simulink model "lateralForceEstimator"  (R2015b)
settings: Solver=FixedStepAuto  StartTime=0.0  StopTime=1.0  FixedStep=0.001  RelTol=1e-3
values from neighbouring files (symbols this model uses):
  Iz = 4605    [ecs.m]
  lf = 1.141    [ecs.m]
  lr = 1.639    [ecs.m]
  mv = 1529.98    [ecs.m]
undefined symbols (not defined in the file or in its folder): d
libraries: simulink x2
settings Model: Creator=ADMIN  LastModifiedBy=ADMIN

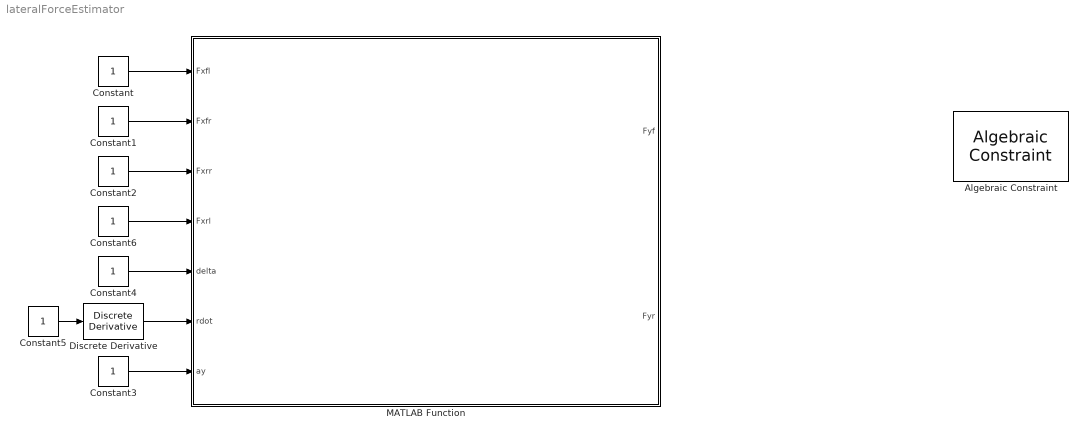
== system lateralForceEstimator ==
  Algebraic Constraint : simulink/Math Operations/Algebraic Constraint  z0=0
  Constant{,1..6} (7 alike) : Constant
  Discrete Derivative : simulink/Discrete/Discrete Derivative  gainval=1.0  ICPrevScaledInput=0.0  InputProcessing=Inherited  OutMin=[]  OutMax=[]  OutDataType=fixdt(1, 16)  OutScaling=2^-10  DoSatur=off
  MATLAB Function : MATLAB Function  InitFcn=|  TreatAsAtomicUnit=on
      | d = 1.795;
      | mv= 1529.98;
      | lf = 1.35;
      | lr = 1.23;
      | Iz = 4605;
  wires:
  Constant/1 -> MATLAB Function/1(Fxfl)
  Constant1/1 -> MATLAB Function/2(Fxfr)
  Constant2/1 -> MATLAB Function/3(Fxrr)
  Constant6/1 -> MATLAB Function/4(Fxrl)
  Constant4/1 -> MATLAB Function/5(delta)
  Constant3/1 -> MATLAB Function/7(ay)
  Constant5/1 -> Discrete Derivative/1
  Discrete Derivative/1 -> MATLAB Function/6(rdot)

== matlab function lateralForceEstimator/MATLAB Function ==
  data: Fxfl input; Fyf output; Fxfr input; Fxrr input; Fxrl input; delta input; rdot input; ay input; Fyr output; d parameter; mv parameter; Iz parameter; lr parameter; lf parameter
function [Fyf, Fyr]= fcn(Fxfl, Fxfr, Fxrr, Fxrl, delta, rdot, ay, d, mv, Iz, lr, lf)
% %#codegen
coder.extrinsic('syms');
syms Fyfs;
syms Fyrs;
% lf * Fyfs * cos(delta) - lr * Fyrs + d/2 * (-Fxfl*cos(delta) + Fxfr*cos(delta)- Fxrl + Fxrr)+ lf*(Fxfl+Fxfr)*sin(delta) - Iz*rdot == 0
[fyf_sol, fyr_sol] = solve(Fxfl*sin(delta) + Fxfr*sin(delta) + Fyfs*cos(delta) + Fyrs - mv*ay == 0, Fyfs, Fyrs);
Fyf = 1;
Fyr = 1;
%Fyf = double(fyf_sol);
%Fyr = double(fyr_sol);
